simulink model "simulacao"  (R2018a)
settings: Solver=VariableStepAuto  StartTime=0.0  StopTime=10000  RelTol=1e-3
libraries: simulink x6
settings Model: Creator=Christopher  LastModifiedBy=Christopher

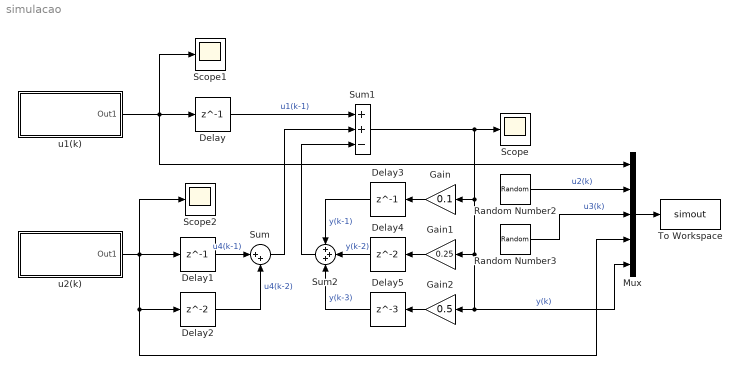
== system simulacao ==
  Delay : Delay  DelayLength=1
  Delay1 : Delay  DelayLength=1
  Delay2 : Delay
  Delay3 : Delay  DelayLength=1
  Delay4 : Delay
  Delay5 : Delay  DelayLength=3
  Gain : Gain  Gain=0.1
  Gain1 : Gain  Gain=0.25
  Gain2 : Gain  Gain=0.5
  Mux : Mux  Inputs=5
  Random Number2 : RandomNumber  Mean=1  Seed=42  SampleTime=50
  Random Number3 : RandomNumber  Mean=5  Variance=2  Seed=3  SampleTime=200
  Scope : Scope
  Scope1 : Scope
  Scope2 : Scope
  Sum : Sum  Inputs=|++
  Sum1 : Sum  Inputs=++-
  Sum2 : Sum  Inputs=+++
  To Workspace : ToWorkspace  VariableName=simout  SampleTime=-1
  u1(k) : Subsystem
  u2(k) : Subsystem
  wires:
  Delay1/1 -> Sum/1  "u4(k-1)"
  Delay2/1 -> Sum/2  "u4(k-2)"
  Delay/1 -> Sum1/1  "u1(k-1)"
  Sum/1 -> Sum1/2
  Sum1/1 -> Scope/1, Mux/5, Gain2/1, Gain1/1, Gain/1  "y(k)"
  Delay3/1 -> Sum2/1  "y(k-1)"
  Delay4/1 -> Sum2/2  "y(k-2)"
  Delay5/1 -> Sum2/3  "y(k-3)"
  Sum2/1 -> Sum1/3
  Mux/1 -> To Workspace/1
  Random Number2/1 -> Mux/2  "u2(k)"
  Random Number3/1 -> Mux/3  "u3(k)"
  Gain/1 -> Delay3/1
  Gain1/1 -> Delay4/1
  Gain2/1 -> Delay5/1
  u1(k)/1(Out1) -> Scope1/1, Mux/1, Delay/1
  u2(k)/1(Out1) -> Mux/4, Delay2/1, Delay1/1, Scope2/1

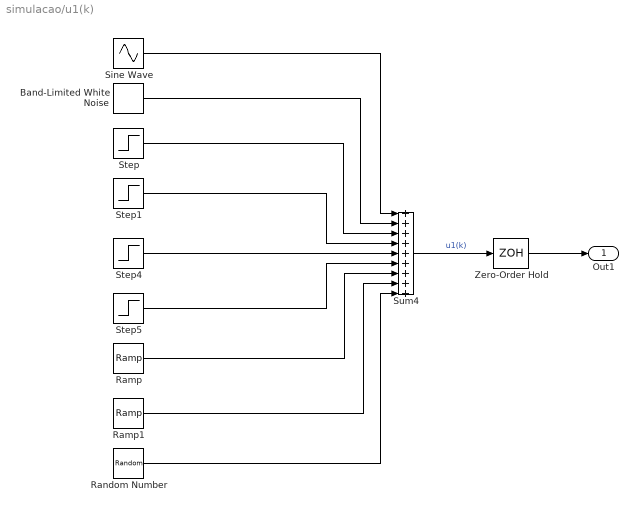
== system simulacao/u1(k) ==
  Band-Limited White Noise : simulink/Sources/Band-Limited White Noise  Cov=[0.005]  Ts=5  seed=[23341]
  Ramp : simulink/Sources/Ramp  slope=0.0003  start=1000  InitialOutput=0
  Ramp1 : simulink/Sources/Ramp  slope=-0.0008  start=5000  InitialOutput=0
  Random Number : RandomNumber  Mean=1  Variance=0.005  Seed=25  SampleTime=250
  Sine Wave : Sin  SineType=Sample based  Amplitude=0.2  Samples=1000  SampleTime=1
  Step : Step  Time=200  After=5  SampleTime=1
  Step1 : Step  Time=5000  After=5  SampleTime=1
  Step4 : Step  Time=2000  After=10  SampleTime=1
  Step5 : Step  Time=8000  After=-3  SampleTime=1
  Sum4 : Sum  Inputs=+++++++++
  Zero-Order Hold : ZeroOrderHold
  Out1 : Outport
  wires:
  Zero-Order Hold/1 -> Out1/1
  Step/1 -> Sum4/3
  Step4/1 -> Sum4/5
  Sine Wave/1 -> Sum4/1
  Random Number/1 -> Sum4/9
  Step5/1 -> Sum4/6
  Sum4/1 -> Zero-Order Hold/1  "u1(k)"
  Step1/1 -> Sum4/4
  Ramp1/1 -> Sum4/8
  Band-Limited White Noise/1 -> Sum4/2
  Ramp/1 -> Sum4/7

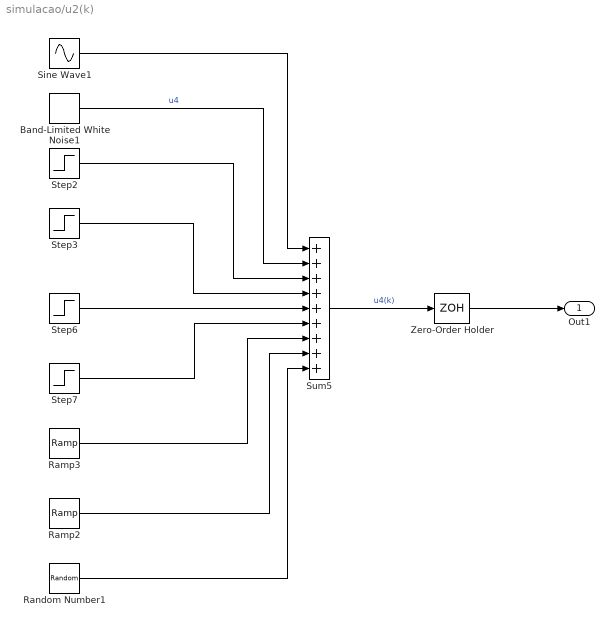
== system simulacao/u2(k) ==
  Band-Limited White Noise1 : simulink/Sources/Band-Limited White Noise  Cov=[0.01]  Ts=5  seed=[333]
  Ramp2 : simulink/Sources/Ramp  slope=0.0005  start=2000  InitialOutput=0
  Ramp3 : simulink/Sources/Ramp  slope=-0.001  start=7000  InitialOutput=0
  Random Number1 : RandomNumber  Mean=0.5  Variance=0.03  Seed=58  SampleTime=300
  Sine Wave1 : Sin  SineType=Sample based  Amplitude=0.1  Samples=700  SampleTime=1  Offset=100
  Step2 : Step  Time=3600  After=-2  SampleTime=1
  Step3 : Step  Time=8000  After=7  SampleTime=1
  Step6 : Step  Time=100  After=3  SampleTime=1
  Step7 : Step  Time=5000  After=-1  SampleTime=1
  Sum5 : Sum  Inputs=+++++++++
  Zero-Order Holder : ZeroOrderHold
  Out1 : Outport
  wires:
  Zero-Order Holder/1 -> Out1/1
  Random Number1/1 -> Sum5/9
  Ramp3/1 -> Sum5/7
  Step6/1 -> Sum5/5
  Band-Limited White Noise1/1 -> Sum5/2  "u4"
  Step7/1 -> Sum5/6
  Sum5/1 -> Zero-Order Holder/1  "u4(k)"
  Sine Wave1/1 -> Sum5/1
  Step2/1 -> Sum5/3
  Step3/1 -> Sum5/4
  Ramp2/1 -> Sum5/8
